simulink model "Step_07"  (Simulink 7.9)
settings: Solver=ode23  StartTime=0.0  StopTime=100  MaxStep=1  RelTol=1e-3
PostLoadFcn:
  | m = 150;
libraries: simulink x1, drag_library_masked x1
settings Model: Creator=wcampbel  LastModifiedBy=wcampbel
settings DebuggingCC: FcnCallInpInsideContextMsg=Use local settings  StrictBusMsg=Warning
settings GRTTargetCC: CombineOutputUpdateFcns=off  GRTInterface=on

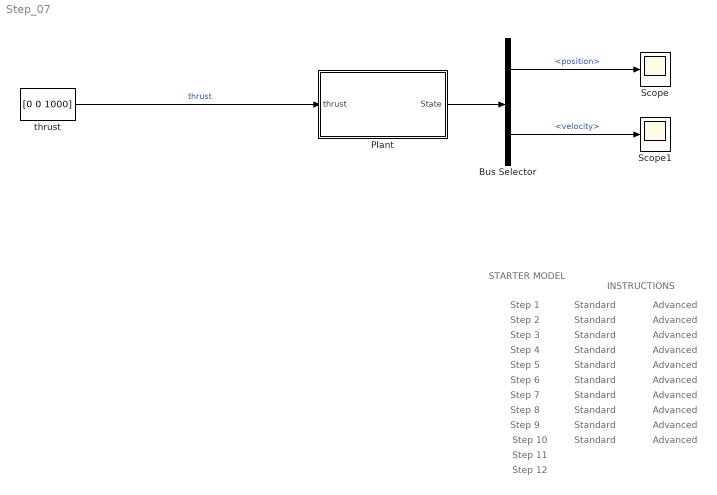
== system Step_07 ==
  note: Step 1
  note: Step 2
  note: Step 3
  note: STARTER
      | MODEL
  note: INSTRUCTIONS
  note: Step 4
  note: Step 5
  note: Step 6
  note: Standard
  note: Advanced
  note: Standard
  note: Advanced
  note: Standard
  note: Advanced
  note: Standard
  note: Standard
  note: Advanced
  note: Standard
  note: Advanced
  note: Step 7
  note: Step 8
  note: Step 9
  note: Step 10
  note: Step 11
  note: Standard
  note: Advanced
  note: Advanced
  note: Advanced
  note: Advanced
  note: Standard
  note: Standard
  note: Standard
  note: Advanced
  note: Step 12
  Bus Selector : BusSelector  OutputSignals=position,velocity
  Plant : Subsystem
  Scope : Scope
      settings: ShowLegends=on  TimeRange=25  YMin=-200  YMax=600
  Scope1 : Scope
      settings: ShowLegends=on  TimeRange=25  YMin=-40  YMax=10
  thrust : Constant  Value=[0 0 1000]
  wires:
  thrust/1 -> Plant/1(thrust)  "thrust"
  Bus Selector/1 -> Scope/1  "<position>"
  Bus Selector/2 -> Scope1/1  "<velocity>"
  Plant/1(State) -> Bus Selector/1

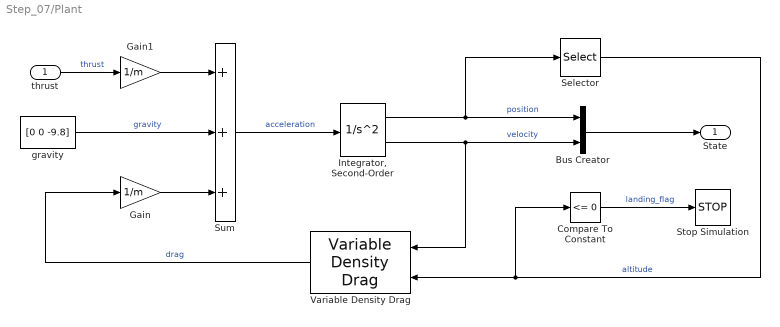
== system Step_07/Plant ==
  thrust : Inport
  Bus Creator : BusCreator  Inputs=2
  Compare To Constant : simulink/Logic and Bit Operations/Compare To Constant  relop=<=  const=0  OutDataTypeStr=boolean
  Gain : Gain  Gain=1/m
  Gain1 : Gain  Gain=1/m
  "Integrator, Second-Order" : SecondOrderIntegrator  ICX=[0 0 500]  ICDXDT=[8 -10 5]
  Selector : Selector  InputPortWidth=3  IndexOptions=Index vector (dialog)  Indices=3  OutputSizes=1
  Stop Simulation : Stop
  Sum : Sum  Inputs=+++
  Variable Density Drag : drag_library_masked/Variable Density Drag  Cd=0.333  A=1.5
  gravity : Constant  Value=[0 0 -9.8]
  State : Outport
  wires:
  "Integrator, Second-Order"/2 -> Variable Density Drag/1, Bus Creator/2  "velocity"
  Variable Density Drag/1 -> Gain/1  "drag"
  Sum/1 -> "Integrator, Second-Order"/1  "acceleration"
  thrust/1 -> Gain1/1  "thrust"
  Gain1/1 -> Sum/1
  gravity/1 -> Sum/2  "gravity"
  Gain/1 -> Sum/3
  Bus Creator/1 -> State/1
  "Integrator, Second-Order"/1 -> Bus Creator/1, Selector/1  "position"
  Selector/1 -> Variable Density Drag/2, Compare To Constant/1  "altitude"
  Compare To Constant/1 -> Stop Simulation/1  "landing_flag"
